simulink model "Navigation_Calculations"  (R2025a)
settings: Solver=FixedStepDiscrete  StartTime=0.0  StopTime=inf  FixedStep=0.001  RelTol=1e-3
settings Model: Creator=deepd  LastModifiedBy=deepd

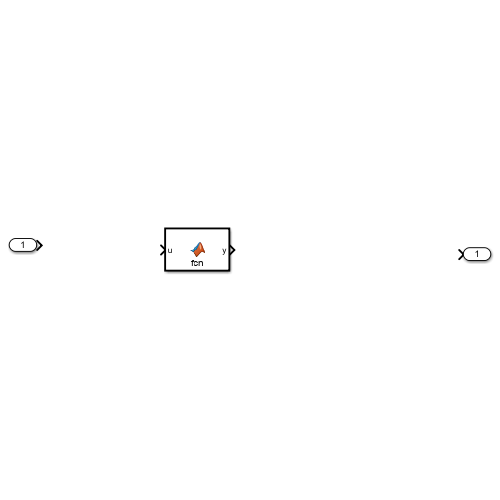
[thumbnail: Simulink's stored preview of the top-level diagram]
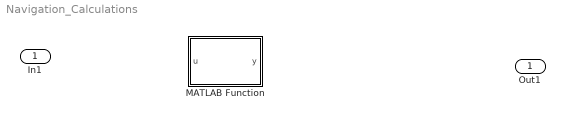
== system Navigation_Calculations ==
  In1 : Inport
  MATLAB Function : MATLAB Function  TreatAsAtomicUnit=on
  Out1 : Outport

== matlab function Navigation_Calculations/MATLAB Function ==
  data: u input; y output
function y = fcn(u)

y = u;
